simulink model "Laengsdynamikmodell_NEmo_MonteCarlo_TestBench"  (R2020b)
settings: Solver=FixedStepAuto  StartTime=0.0  StopTime=1477  FixedStep=0.01  RelTol=1e-3
model workspace (MAT data in the model file):
  C_RR = 0.0103682470085
  SampleTime = 0.01
  StopTime = 1477
  UncertaintyRollerDynamometer = 0.796984855506
  VehMass = 929
  c_w = 0.37
  cycle : timeseries (value not decoded)
  i_gear = 5.6813
  p = 2.5
  power_map_LE = [81.3594367777 81.3594367777 88.9151238368 69.3920543425 121.856227925 33.5913037104 56.5214963128 60.6342218487 61.1595876762 53.4292335319 53.4133899816 35.6771556802 ... (16260 elements, 60x271)]
  power_map_Mot = [0 74.834999341 40.2428359465 95.3690451807 75.6091573236 114.707467852 143.074401876 144.922747771 177.284289075 184.351766643 192.404587732 197.413952644 ... (16260 elements, 60x271)]
  r_dyn = 0.275233869952
undefined symbols (not defined in the file): DiscIntNeverNeededParam, gravity, UncertaintyMappedLosses, UncertaintyTabledConsumption, v_HA
libraries: Constant_Environment x1, Driver_PI x1, Longitudinal_DrivingCycles x1, Acceleration_Calculation x1, Air_Resistance x1, Roll_Resistance x1, Slope_Resistance x1, Simple_Auxiliary x1, Electric_Drive_Tabled_Consumption x1, Gear_Stage x1, DCAC_Converter x1, Control_Unit_Simple x1
(part 3 of 3)

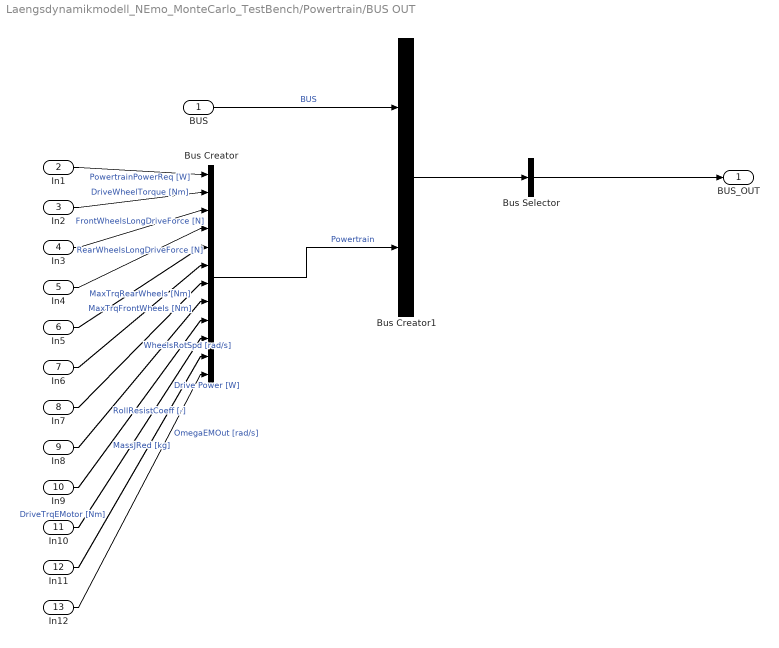
== system Laengsdynamikmodell_NEmo_MonteCarlo_TestBench/Powertrain/BUS OUT ==
  BUS : Inport
  In1 : Inport  Port=2
  In2 : Inport  Port=3
  In3 : Inport  Port=4
  In4 : Inport  Port=5
  In5 : Inport  Port=6
  In6 : Inport  Port=7
  In7 : Inport  Port=8
  In8 : Inport  Port=9
  In9 : Inport  Port=10
  In10 : Inport  Port=11
  In11 : Inport  Port=12
  In12 : Inport  Port=13
  Bus Creator : BusCreator  Inputs=12
  Bus Creator1 : BusCreator  Inputs=2
  Bus Selector : BusSelector  OutputSignals=Powertrain,BUS.Powersource,BUS.VehicleControlUnit,BUS.Driver and Enironment,BUS.DrivinCycle,BUS.Bus_Old  OutputAsBus=on
  BUS_OUT : Outport  VectorParamsAs1DForOutWhenUnconnected=off
  wires:
  Bus Creator1/1 -> Bus Selector/1
  BUS/1 -> Bus Creator1/1  "BUS"
  Bus Creator/1 -> Bus Creator1/2  "Powertrain"
  Bus Selector/1 -> BUS_OUT/1
  In1/1 -> Bus Creator/1  "PowertrainPowerReq [W]"
  In2/1 -> Bus Creator/2  "DriveWheelTorque [Nm]"
  In3/1 -> Bus Creator/3  "FrontWheelsLongDriveForce [N]"
  In4/1 -> Bus Creator/4  "RearWheelsLongDriveForce [N]"
  In5/1 -> Bus Creator/5  "MaxTrqRearWheels [Nm]"
  In6/1 -> Bus Creator/6  "MaxTrqFrontWheels [Nm]"
  In7/1 -> Bus Creator/7  "WheelsRotSpd [rad/s]"
  In8/1 -> Bus Creator/8  "RollResistCoeff [-]"
  In9/1 -> Bus Creator/9  "MassJRed [kg]"
  In10/1 -> Bus Creator/10  "Drive Power [W]"
  In11/1 -> Bus Creator/11  "DriveTrqEMotor [Nm]"
  In12/1 -> Bus Creator/12  "OmegaEMOut [rad/s]"

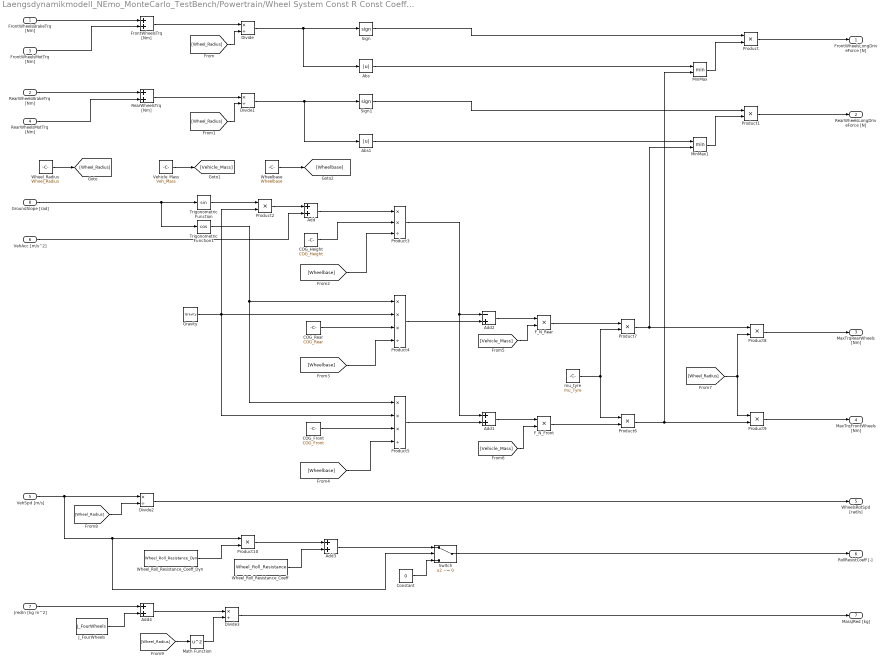
== system Laengsdynamikmodell_NEmo_MonteCarlo_TestBench/Powertrain/Wheel System Const R Const Coefficient ==
  FrontWheelsBrakeTrq [Nm] : Inport  SampleTime=LocalSampleTime
  RearWheelsBrakeTrq [Nm] : Inport  Port=2  SampleTime=LocalSampleTime
  FrontWheelsMotTrq [Nm] : Inport  Port=3  SampleTime=LocalSampleTime
  RearWheelsMotTrq [Nm] : Inport  Port=4  SampleTime=LocalSampleTime
  VehSpd [m/s] : Inport  Port=5  SampleTime=LocalSampleTime
  VehAcc [m/s^2] : Inport  Port=6  SampleTime=LocalSampleTime
  JredIn [kg m^2] : Inport  Port=7  SampleTime=LocalSampleTime
  GroundSlope [rad] : Inport  Port=8  SampleTime=LocalSampleTime
  Abs : Abs
  Abs1 : Abs
  Add{,1,3..4} (4 alike) : Sum
  Add2 : Sum  Inputs=-+
  COG_Front : Constant  Value=COG_Front
  COG_Height : Constant  Value=COG_Height
  COG_Rear : Constant  Value=COG_Rear
  Constant : Constant  Value=0
  Divide{,1..3} (4 alike) : Product  Inputs=*/
  F_N_Front : Product
  F_N_Rear : Product
  FrontWheelsTrq [Nm] : Sum
  Gravity : Constant  Value=Gravity
  J_FourWheels : Constant  Value=J_FourWheels
  Math Function : Math  Operator=square  SignedPower=on  SaturateOnIntegerOverflow=on
  MinMax : MinMax  Inputs=2
  MinMax1 : MinMax  Inputs=2
  Product{,1..2,6..10} (8 alike) : Product
  Product3 : Product  Inputs=**/
  Product4 : Product  Inputs=***/
  Product5 : Product  Inputs=***/
  RearWheelsTrq [Nm] : Sum
  Sign : Signum
  Sign1 : Signum
  Switch : Switch  Criteria=u2 ~= 0
  Trigonometric Function : Trigonometry
  Trigonometric Function1 : Trigonometry  Operator=cos
  Vehicle_Mass : Constant  Value=Veh_Mass
  Wheel_Radius : Constant  Value=Wheel_Radius
  Wheel_Roll_Resistance_Coeff : Constant  Value=Wheel_Roll_Resistance
  Wheel_Roll_Resistance_Coeff_Dyn : Constant  Value=Wheel_Roll_Resistance_Dyn
  Wheelbase : Constant  Value=Wheelbase
  mu_tyre : Constant  Value=mu_Tyre
  FrontWheelsLongDriveForce [N] : Outport  SampleTime=GlobalSampleTime  VectorParamsAs1DForOutWhenUnconnected=off
  RearWheelsLongDriveForce [N] : Outport  Port=2  SampleTime=GlobalSampleTime  VectorParamsAs1DForOutWhenUnconnected=off
  MaxTrqRearWheels [Nm] : Outport  Port=3  SampleTime=GlobalSampleTime  VectorParamsAs1DForOutWhenUnconnected=off
  MaxTrqFrontWheels [Nm] : Outport  Port=4  SampleTime=GlobalSampleTime  VectorParamsAs1DForOutWhenUnconnected=off
  WheelsRotSpd [rad/s] : Outport  Port=5  SampleTime=GlobalSampleTime  VectorParamsAs1DForOutWhenUnconnected=off
  RollResistCoeff [-] : Outport  Port=6  SampleTime=GlobalSampleTime  VectorParamsAs1DForOutWhenUnconnected=off
  MassJRed [kg] : Outport  Port=7  SampleTime=GlobalSampleTime  VectorParamsAs1DForOutWhenUnconnected=off
  wires:
  Divide3/1 -> MassJRed [kg]/1
  [Wheel_Radius] -> Math Function/1
  Math Function/1 -> Divide3/2
  Add4/1 -> Divide3/1
  J_FourWheels/1 -> Add4/2
  JredIn [kg m^2]/1 -> Add4/1
  Switch/1 -> RollResistCoeff [-]/1
  Constant/1 -> Switch/3
  Add3/1 -> Switch/1
  Wheel_Roll_Resistance_Coeff/1 -> Add3/2
  Product10/1 -> Add3/1
  Wheel_Roll_Resistance_Coeff_Dyn/1 -> Product10/2
  Divide2/1 -> WheelsRotSpd [rad/s]/1
  [Wheel_Radius] -> Divide2/2
  VehSpd [m/s]/1 -> Divide2/1, Product10/1, Switch/2
  Product9/1 -> MaxTrqFrontWheels [Nm]/1
  Product8/1 -> MaxTrqRearWheels [Nm]/1
  [Wheel_Radius] -> Product9/1, Product8/2
  Product7/1 -> MinMax1/2, Product8/1
  Product6/1 -> MinMax/2, Product9/2
  mu_tyre/1 -> Product7/2, Product6/1
  F_N_Front/1 -> Product6/2
  F_N_Rear/1 -> Product7/1
  [Vehicle_Mass] -> F_N_Front/2
  [Vehicle_Mass] -> F_N_Rear/2
  Add1/1 -> F_N_Front/1
  Add2/1 -> F_N_Rear/1
  Product4/1 -> Add2/2
  Product3/1 -> Add1/1, Add2/1
  Product5/1 -> Add1/2
  [Wheelbase] -> Product5/4
  COG_Front/1 -> Product5/3
  [Wheelbase] -> Product4/4
  [Wheelbase] -> Product3/3
  Wheelbase/1 -> [Wheelbase]
  COG_Rear/1 -> Product4/3
  Gravity/1 -> Product4/2, Product5/2, Product2/2
  Trigonometric Function1/1 -> Product5/1, Product4/1
  COG_Height/1 -> Product3/2
  Add/1 -> Product3/1
  VehAcc [m/s^2]/1 -> Add/2
  Product2/1 -> Add/1
  Trigonometric Function/1 -> Product2/1
  GroundSlope [rad]/1 -> Trigonometric Function/1, Trigonometric Function1/1
  Vehicle_Mass/1 -> [Vehicle_Mass]
  Product1/1 -> RearWheelsLongDriveForce [N]/1
  MinMax1/1 -> Product1/2
  Sign1/1 -> Product1/1
  Abs1/1 -> MinMax1/1
  Divide1/1 -> Sign1/1, Abs1/1
  [Wheel_Radius] -> Divide1/2
  [Wheel_Radius] -> Divide/2
  Wheel_Radius/1 -> [Wheel_Radius]
  MinMax/1 -> Product/2
  Abs/1 -> MinMax/1
  Divide/1 -> Sign/1, Abs/1
  Sign/1 -> Product/1
  Product/1 -> FrontWheelsLongDriveForce [N]/1
  RearWheelsTrq [Nm]/1 -> Divide1/1
  FrontWheelsTrq [Nm]/1 -> Divide/1
  RearWheelsMotTrq [Nm]/1 -> RearWheelsTrq [Nm]/2
  RearWheelsBrakeTrq [Nm]/1 -> RearWheelsTrq [Nm]/1
  FrontWheelsMotTrq [Nm]/1 -> FrontWheelsTrq [Nm]/2
  FrontWheelsBrakeTrq [Nm]/1 -> FrontWheelsTrq [Nm]/1

== system Laengsdynamikmodell_NEmo_MonteCarlo_TestBench/Results/BUS IN ==
  BUS_In : Inport
  Bus Selector : BusSelector  OutputSignals=DrivinCycle.v [m/s],Dynamics.VehSpd [m/s],Dynamics.VehPos [m],Powersource.ActualPower [W],Powertrain.DriveWheelTorque [Nm]
  BUS : Outport  VectorParamsAs1DForOutWhenUnconnected=off
  v [m/s] : Outport  Port=2  VectorParamsAs1DForOutWhenUnconnected=off
  VehSpd [m/s] : Outport  Port=3  VectorParamsAs1DForOutWhenUnconnected=off
  VehPos [m] : Outport  Port=4  VectorParamsAs1DForOutWhenUnconnected=off
  ActualPower [W] : Outport  Port=5  VectorParamsAs1DForOutWhenUnconnected=off
  DriveWheelTorque [Nm] : Outport  Port=6  VectorParamsAs1DForOutWhenUnconnected=off
  wires:
  BUS_In/1 -> BUS/1, Bus Selector/1
  Bus Selector/1 -> v [m/s]/1  "<v [m/s]>"
  Bus Selector/2 -> VehSpd [m/s]/1  "<VehSpd [m/s]>"
  Bus Selector/3 -> VehPos [m]/1  "<VehPos [m]>"
  Bus Selector/4 -> ActualPower [W]/1  "<ActualPower [W]>"
  Bus Selector/5 -> DriveWheelTorque [Nm]/1  "<DriveWheelTorque [Nm]>"

== system Laengsdynamikmodell_NEmo_MonteCarlo_TestBench/Results/Subsystem ==
  Actual power Power Source [W] : Inport
  Discrete-Time Integrator : DiscreteIntegrator  SampleTime=-1  ICPrevOutput=DiscIntNeverNeededParam  ICPrevScaledInput=DiscIntNeverNeededParam
  Gain1 : Gain  Gain=1/3600
  CumulativeConsumption [Wh] : Outport  Unit=W*h
  wires:
  Discrete-Time Integrator/1 -> Gain1/1
  Gain1/1 -> CumulativeConsumption [Wh]/1  "CumulativeConsumption [Wh]"
  Actual power Power Source [W]/1 -> Discrete-Time Integrator/1

== system Laengsdynamikmodell_NEmo_MonteCarlo_TestBench/Vehicle Control Unit/BUS IN ==
  BUS_In : Inport
  Bus Selector : BusSelector  OutputSignals=Driver and Enironment.AccPedalPos [-],Driver and Enironment.BrakePedalPos [-]
  BUS : Outport  VectorParamsAs1DForOutWhenUnconnected=off
  AccPedalPos [-] : Outport  Port=2  VectorParamsAs1DForOutWhenUnconnected=off
  BrakePedalPos [-] : Outport  Port=3  VectorParamsAs1DForOutWhenUnconnected=off
  wires:
  BUS_In/1 -> Bus Selector/1, BUS/1
  Bus Selector/1 -> AccPedalPos [-]/1  "<AccPedalPos [-]>"
  Bus Selector/2 -> BrakePedalPos [-]/1  "<BrakePedalPos [-]>"

== system Laengsdynamikmodell_NEmo_MonteCarlo_TestBench/Vehicle Control Unit/BUS OUT ==
  BUS : Inport
  In1 : Inport  Port=2
  In2 : Inport  Port=3
  In3 : Inport  Port=4
  Bus Creator : BusCreator  Inputs=3
  Bus Creator1 : BusCreator  Inputs=2
  Bus Selector : BusSelector  OutputSignals=VehicleControlUnit,BUS.Driver and Enironment,BUS.DrivinCycle,BUS.Bus_Old  OutputAsBus=on
  BUS_OUT : Outport  VectorParamsAs1DForOutWhenUnconnected=off
  wires:
  Bus Creator1/1 -> Bus Selector/1
  BUS/1 -> Bus Creator1/1  "BUS"
  Bus Creator/1 -> Bus Creator1/2  "VehicleControlUnit"
  Bus Selector/1 -> BUS_OUT/1
  In1/1 -> Bus Creator/1  "TargetDriveTrq [Nm]"
  In2/1 -> Bus Creator/2  "TargetBrakeTrqFrontAxle [Nm]"
  In3/1 -> Bus Creator/3  "TargetBrakeTrqRearAxle [Nm]"
